simulink library "ahlb"  (Simulink 8.2)
settings: Solver=ode1  StartTime=0.0  StopTime=Inf  FixedStep=0.001  RelTol=1e-3
PostLoadFcn:
  | , if any(exist('dsrtsu_mdlpostloadfcn', 'file') == [2, 3, 6]), try dsrtsu_mdlpostloadfcn('Execute', bdroot); catch fprintf('Error in PostLoadFcn (dsrtsu_mdlpostloadfcn) for model "%s":\n %s\n', bdroot, lasterr); end, end,
undefined symbols (not defined in the file or in its folder): KAHLB_HighBeamTimeHighLimit_s, KAHLB_HighBeamTimeLowLimit_s, KAHLB_NoObjectTimeHighLimit_s, KAHLB_NoObjectTimeLowLimit_s
libraries: simulink x2
settings Model: DSRTSU_INTERNAL_RTI_VER=440  DSRTSU_INTERNAL_RTI_TYPE=rti1401  RTICANMMDATA=struct('GeneralSetupData',struct('modelroot','D:\HAITEC\SVN\trunk\ADAS_Softwares\HTDragon\software\sw_development\arch\app\ahlb','generalsettings',struct('filesettings',struct('destfolder',struct('Name','RTICANMM_FILES','Check',1),'buildfolder',struct('Name','.','Check',1),'AbsDestfolder',struct('Name','D:\HAITEC\SVN\trunk\ADAS_Softwares\HTDragon\software\sw_development\arch\app\ahlb\RTICANMM_FILES'),'AbsBuildfolder',struct('Name','D:\HAITEC\SVN\trunk\ADAS_Softwares\HTDragon\software\sw_development\arch\app\ahlb'))),'options',struct('addpaths',1,'rmpaths',1,'addtrcexclusion',logical(1),'cannavigator',struct('checkmonitoring',0),'show_usrtrc',0,'use_usrtrc',0),'advanced',struct('options',[1 1 1 1 1 1 1 1 1 1 1 1 1 1 1 1 1 1 1 1 1 1 1 1 1 1 1 1 1 1 1 1 1 1 1 1 1 1 1 1 1 1 1 1 1 1 1 1 1 1 1 1 1 1 1 1 1 1 1 1 1 1 1 1 1 1 1 1 1 1 1 1 1 1 1 1 1 1 1 1 1 1 1 1 1 1 1 1 1 1 1 1 1 1 1 1 1 1 1 1]),'MPSetup',{{}},'modelname','ahlb','block','ahlb'))  DSRTSU_INTERNAL_RTIFPGA=30  Creator=14014  LastModifiedBy=14014

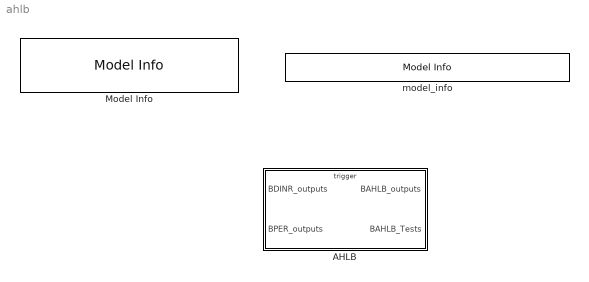
== system ahlb ==
  AHLB : Subsystem
      settings: RTWSystemCode=Nonreusable function  RTWFcnNameOpts=Use subsystem name  RTWFileNameOpts=Use subsystem name
  Model Info : simulink/Model-Wide Utilities/Model Info  InitialBlockCM=None  BlockCM=None  Frame=on  DisplayStringWithTags=|  HorizontalTextAlignment=Left  LeftAlignmentValue=0.02  SourceBlockDiagram=ahlb  TagMaxNumber=20
      | Model Version        : %<ModelVersion>
      | Creator                   : %<Creator>
      | Last Modified by    : %<LastModifiedBy>
  model_info : simulink/Model-Wide Utilities/Model Info  InitialBlockCM=None  BlockCM=None  Frame=on  DisplayStringWithTags=$Id: ahlb.mdl 1419 2016-06-27 04:04:52Z chimotsai $  HorizontalTextAlignment=Center  LeftAlignmentValue=0.5  SourceBlockDiagram=ahlb  TagMaxNumber=20

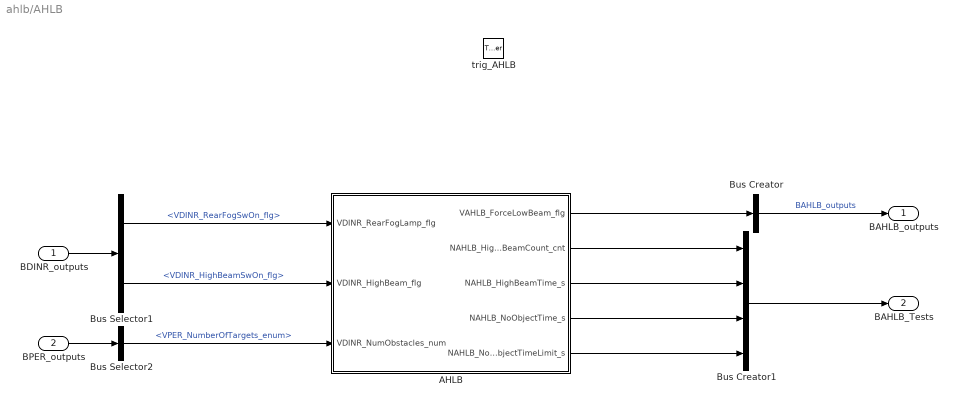
== system ahlb/AHLB ==
  BDINR_outputs : Inport  OutDataTypeStr=Bus: BDINR_outputs
  BPER_outputs : Inport  Port=2  OutDataTypeStr=Bus: BPER_outputs
  trig_AHLB : TriggerPort  TriggerType=function-call
  AHLB : Subsystem
  Bus Creator : BusCreator  Inputs=1  OutDataTypeStr=Bus: BAHLB_outputs
  Bus Creator1 : BusCreator
  Bus Selector1 : BusSelector  OutputSignals=VDINR_RearFogSwOn_flg,VDINR_HighBeamSwOn_flg
  Bus Selector2 : BusSelector  OutputSignals=VPER_NumberOfTargets_enum
  BAHLB_outputs : Outport  OutDataTypeStr=Bus: BAHLB_outputs
  BAHLB_Tests : Outport  Port=2
  wires:
  AHLB/1(VAHLB_ForceLowBeam_flg) -> Bus Creator/1
  Bus Creator/1 -> BAHLB_outputs/1  "BAHLB_outputs"
  BDINR_outputs/1 -> Bus Selector1/1
  Bus Selector1/1 -> AHLB/1(VDINR_RearFogLamp_flg)  "<VDINR_RearFogSwOn_flg>"
  Bus Selector1/2 -> AHLB/2(VDINR_HighBeam_flg)  "<VDINR_HighBeamSwOn_flg>"
  BPER_outputs/1 -> Bus Selector2/1
  Bus Selector2/1 -> AHLB/3(VDINR_NumObstacles_num)  "<VPER_NumberOfTargets_enum>"
  AHLB/2(NAHLB_HighBeamCount_cnt) -> Bus Creator1/1
  AHLB/3(NAHLB_HighBeamTime_s) -> Bus Creator1/2
  AHLB/4(NAHLB_NoObjectTime_s) -> Bus Creator1/3
  AHLB/5(NAHLB_NoObjectTimeLimit_s) -> Bus Creator1/4
  Bus Creator1/1 -> BAHLB_Tests/1

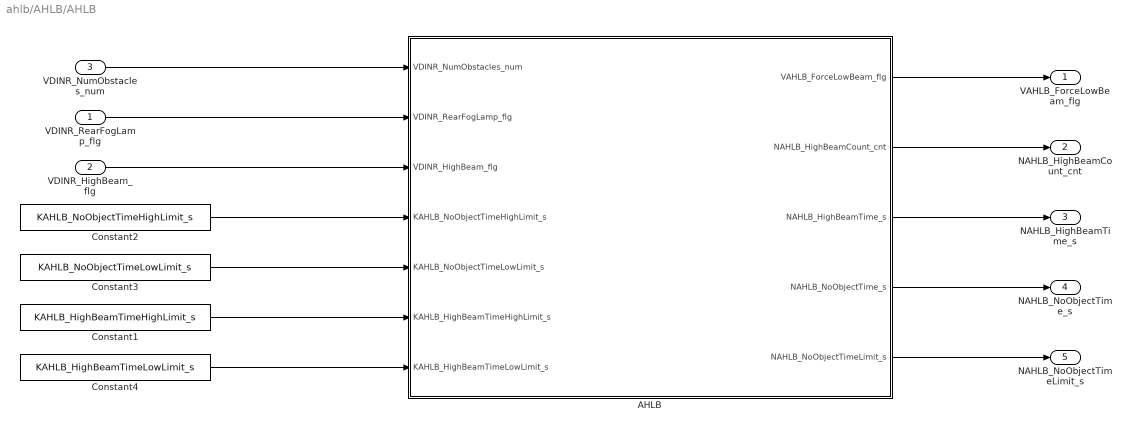
== system ahlb/AHLB/AHLB ==
  VDINR_RearFogLamp_flg : Inport
  VDINR_HighBeam_flg : Inport  Port=2
  VDINR_NumObstacles_num : Inport  Port=3
  AHLB : Stateflow chart  TreatAsAtomicUnit=on
  Constant1 : Constant  Value=KAHLB_HighBeamTimeHighLimit_s
  Constant2 : Constant  Value=KAHLB_NoObjectTimeHighLimit_s
  Constant3 : Constant  Value=KAHLB_NoObjectTimeLowLimit_s
  Constant4 : Constant  Value=KAHLB_HighBeamTimeLowLimit_s
  VAHLB_ForceLowBeam_flg : Outport
  NAHLB_HighBeamCount_cnt : Outport  Port=2
  NAHLB_HighBeamTime_s : Outport  Port=3
  NAHLB_NoObjectTime_s : Outport  Port=4
  NAHLB_NoObjectTimeLimit_s : Outport  Port=5
  wires:
  Constant4/1 -> AHLB/7(KAHLB_HighBeamTimeLowLimit_s)
  Constant1/1 -> AHLB/6(KAHLB_HighBeamTimeHighLimit_s)
  Constant3/1 -> AHLB/5(KAHLB_NoObjectTimeLowLimit_s)
  AHLB/1(VAHLB_ForceLowBeam_flg) -> VAHLB_ForceLowBeam_flg/1
  Constant2/1 -> AHLB/4(KAHLB_NoObjectTimeHighLimit_s)
  VDINR_NumObstacles_num/1 -> AHLB/1(VDINR_NumObstacles_num)
  VDINR_RearFogLamp_flg/1 -> AHLB/2(VDINR_RearFogLamp_flg)
  VDINR_HighBeam_flg/1 -> AHLB/3(VDINR_HighBeam_flg)
  AHLB/2(NAHLB_HighBeamCount_cnt) -> NAHLB_HighBeamCount_cnt/1
  AHLB/3(NAHLB_HighBeamTime_s) -> NAHLB_HighBeamTime_s/1
  AHLB/4(NAHLB_NoObjectTime_s) -> NAHLB_NoObjectTime_s/1
  AHLB/5(NAHLB_NoObjectTimeLimit_s) -> NAHLB_NoObjectTimeLimit_s/1

== stateflow chart AHLB/AHLB/AHLB ==
  state DISABLE
    en:
    VAHLB_ForceLowBeam_flg=0;
    NAHLB_HighBeamCount_cnt=0;
    NAHLB_NoObjectTimeLimit_s=...
    KAHLB_NoObjectTimeLowLimit_s;
  state ENABLE
    state LOW_BEAM
      en:
      VAHLB_ForceLowBeam_flg=0;
      NAHLB_HighBeamTime_s=C_TASK_5MS_S;
      du:
      NAHLB_HighBeamTime_s=NAHLB_HighBeamTime_s+C_TASK_5MS_S;
    state HIGH_BEAM
      en:
      VAHLB_ForceLowBeam_flg=1;
      state SELECT_DELAY_TIME
        (default) -> (junction 10)
        (junction 10) -> (junction 11) [order 1] : [NAHLB_HighBeamTime_s <= KAHLB_HighBeamTimeLowLimit_s]
        (junction 10) -> (junction 12) [order 2] : {
            | NAHLB_HighBeamCount_cnt=0;
            | }
        (junction 11) -> (junction 13) : {
            | NAHLB_HighBeamCount_cnt = NAHLB_HighBeamCount_cnt+1;
            | }
        (junction 13) -> (junction 12) [order 2]
        (junction 13) -> (junction 14) [order 1] : [NAHLB_HighBeamCount_cnt >= 3]
        (junction 12) -> (junction 15)
        (junction 14) -> (junction 16) : {
            | NAHLB_NoObjectTimeLimit_s = KAHLB_NoObjectTimeHighLimit_s;
            | }
        (junction 16) -> (junction 15)
        (junction 15) -> (junction 17)
        (junction 17) -> (junction 18) [order 1] : [NAHLB_HighBeamTime_s >= KAHLB_HighBeamTimeHighLimit_s]
        (junction 18) -> (junction 20) : {
            | NAHLB_NoObjectTimeLimit_s = KAHLB_NoObjectTimeLowLimit_s;
            | }
        (junction 17) -> (junction 19) [order 2]
        (junction 20) -> (junction 19)
      state NO_OBJECTS
        du:
        NAHLB_NoObjectTime_s=NAHLB_NoObjectTime_s+C_TASK_5MS_S;
      state HAVE_OBJECTS
        en:
        NAHLB_NoObjectTime_s=C_TASK_5MS_S;
      (default) -> SELECT_DELAY_TIME
      HAVE_OBJECTS -> NO_OBJECTS : [VDINR_NumObstacles_num==0]
      SELECT_DELAY_TIME -> HAVE_OBJECTS
      NO_OBJECTS -> HAVE_OBJECTS : [VDINR_NumObstacles_num>0]
    (default) -> LOW_BEAM
    LOW_BEAM -> HIGH_BEAM : [VDINR_NumObstacles_num > 0]
    HIGH_BEAM -> LOW_BEAM : [NAHLB_NoObjectTime_s >= NAHLB_NoObjectTimeLimit_s...
        | &&VDINR_NumObstacles_num==0]
  (default) -> DISABLE
  DISABLE -> ENABLE : [VDINR_RearFogLamp_flg && VDINR_HighBeam_flg]
  ENABLE -> DISABLE : [!VDINR_RearFogLamp_flg || !VDINR_HighBeam_flg]
  data: VDINR_NumObstacles_num input double; VAHLB_ForceLowBeam_flg output double; VDINR_RearFogLamp_flg input double; VDINR_HighBeam_flg input double; KAHLB_NoObjectTimeHighLimit_s input double; KAHLB_NoObjectTimeLowLimit_s input double; KAHLB_HighBeamTimeHighLimit_s input double; KAHLB_HighBeamTimeLowLimit_s input double; NAHLB_HighBeamCount_cnt output uint8; NAHLB_HighBeamTime_s output single; NAHLB_NoObjectTime_s output single; NAHLB_NoObjectTimeLimit_s output single; C_TASK_5MS_S parameter double
